simulink model "Aula7_3"  (R2013b)
settings: Solver=ode45  StartTime=0.0  StopTime=10  RelTol=1e-3
settings Model: Creator=ThiagoCordeiro  LastModifiedBy=ThiagoFelippe

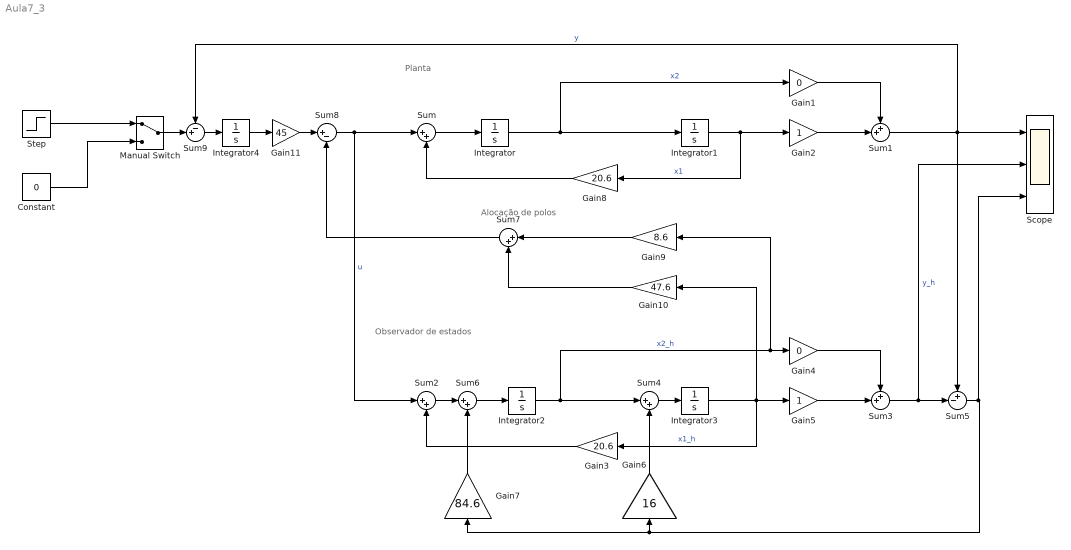
== system Aula7_3 ==
  note: Alocação de polos
  note: Planta
  note: Observador de estados
  Constant : Constant  Value=0
  Gain1 : Gain  Gain=0
  Gain10 : Gain  Gain=47.6
  Gain11 : Gain  Gain=45
  Gain2 : Gain
  Gain3 : Gain  Gain=20.6
  Gain4 : Gain  Gain=0
  Gain5 : Gain
  Gain6 : Gain  Gain=16
  Gain7 : Gain  Gain=84.6
  Gain8 : Gain  Gain=20.6
  Gain9 : Gain  Gain=8.6
  Integrator : Integrator  InitialCondition=5
  Integrator1 : Integrator  InitialCondition=2
  Integrator2 : Integrator
  Integrator3 : Integrator
  Integrator4 : Integrator
  Manual Switch : ManualSwitch
  Scope : Scope  NumInputPorts=3
      settings: YMin=-5~-5~-5  YMax=5~5~5
  Step : Step  SampleTime=0
  Sum{,2,4,6..7} (5 alike) : Sum  Inputs=|++
  Sum1 : Sum  Inputs=++|
  Sum3 : Sum  Inputs=++|
  Sum5 : Sum  Inputs=+-|
  Sum8 : Sum  Inputs=|+-
  Sum9 : Sum  Inputs=-+|
  wires:
  Step/1 -> Manual Switch/1
  Sum/1 -> Integrator/1
  Constant/1 -> Manual Switch/2
  Integrator/1 -> Integrator1/1, Gain1/1  "x2"
  Integrator1/1 -> Gain8/1, Gain2/1  "x1"
  Gain2/1 -> Sum1/2
  Gain1/1 -> Sum1/1
  Sum1/1 -> Sum9/1, Sum5/1, Scope/1  "y"
  Integrator2/1 -> Sum4/1, Gain9/1, Gain4/1  "x2_h"
  Integrator3/1 -> Gain10/1, Gain3/1, Gain5/1  "x1_h"
  Gain5/1 -> Sum3/2
  Gain4/1 -> Sum3/1
  Sum3/1 -> Scope/2, Sum5/2  "y_h"
  Sum4/1 -> Integrator3/1
  Gain6/1 -> Sum4/2
  Sum5/1 -> Scope/3, Gain7/1, Gain6/1
  Sum2/1 -> Sum6/1
  Sum6/1 -> Integrator2/1
  Gain7/1 -> Sum6/2
  Gain8/1 -> Sum/2
  Gain3/1 -> Sum2/2
  Gain9/1 -> Sum7/1
  Gain10/1 -> Sum7/2
  Sum7/1 -> Sum8/2
  Sum8/1 -> Sum2/1, Sum/1  "u"
  Manual Switch/1 -> Sum9/2
  Sum9/1 -> Integrator4/1
  Integrator4/1 -> Gain11/1
  Gain11/1 -> Sum8/1
